simulink model "probs6"  (R2020b)
settings: Solver=FixedStepAuto  StartTime=0.0  StopTime=100.0  FixedStep=2  RelTol=1e-3
settings Model: Creator=gokul  LastModifiedBy=gokul
settings DataIOCC: SaveOutput=off  SaveTime=off

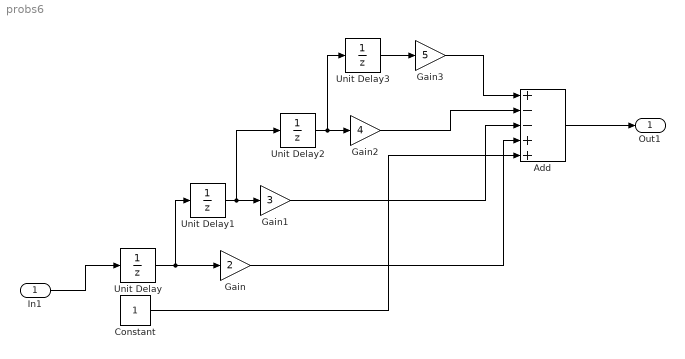
== system probs6 ==
  In1 : Inport  OutDataTypeStr=double  PortDimensions=1  SampleTime=[0,1]
  Add : Sum  Inputs=+--++
  Constant : Constant
  Gain : Gain  Gain=2
  Gain1 : Gain  Gain=3
  Gain2 : Gain  Gain=4
  Gain3 : Gain  Gain=5
  Unit Delay{,1..3} (4 alike) : UnitDelay  SampleTime=-1  HasFrameUpgradeWarning=on
  Out1 : Outport  OutDataTypeStr=double  PortDimensions=1  SampleTime=[2,0]
  wires:
  Constant/1 -> Add/5
  Unit Delay1/1 -> Gain1/1, Unit Delay2/1
  In1/1 -> Unit Delay/1
  Unit Delay/1 -> Gain/1, Unit Delay1/1
  Gain3/1 -> Add/1
  Gain/1 -> Add/4
  Unit Delay2/1 -> Gain2/1, Unit Delay3/1
  Gain2/1 -> Add/2
  Unit Delay3/1 -> Gain3/1
  Gain1/1 -> Add/3
  Add/1 -> Out1/1
